simulink model "ITMBS_epushbtton_M1_Test_Harness"  (R2023a)
settings: Solver=FixedStepDiscrete  StartTime=0.0  StopTime=10  FixedStep=0.05  RelTol=1e-3
undefined symbols (not defined in the file or in its folder): sigbuilder_block
libraries: legoev3lib x2
settings Model: Creator=kevin  LastModifiedBy=Sachin K S

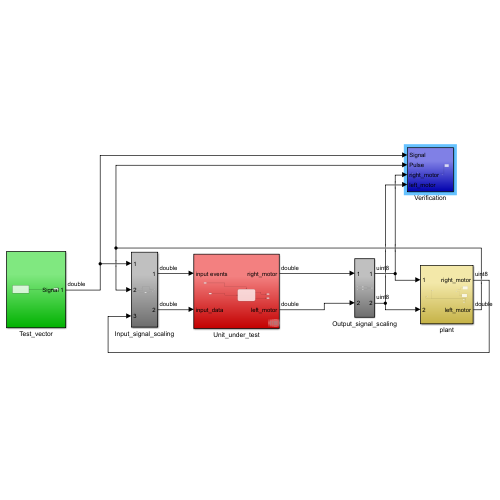
[thumbnail: Simulink's stored preview of the top-level diagram]
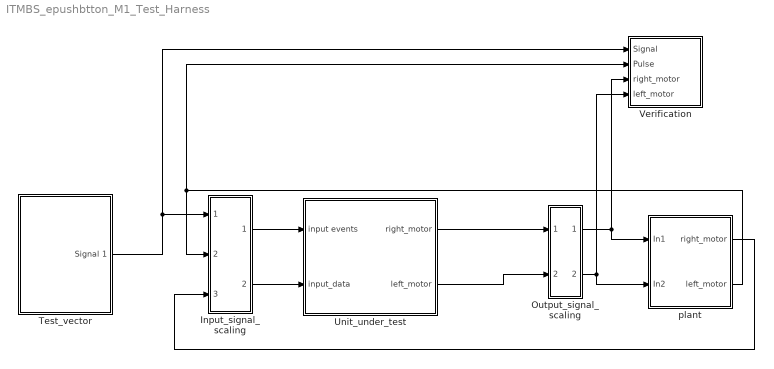
== system ITMBS_epushbtton_M1_Test_Harness ==
  Input_signal_scaling : Subsystem
  Output_signal_scaling : Subsystem
  Test_vector : Subsystem
  Unit_under_test : Subsystem
  Verification : Subsystem
  plant : Subsystem
  wires:
  Test_vector/1(Signal 1) -> Verification/1(Signal), Input_signal_scaling/1(In1)
  Unit_under_test/1(right_motor) -> Output_signal_scaling/1(In1)
  Output_signal_scaling/1(Out1) -> plant/1(In1), Verification/3(right_motor)
  plant/1(right_motor) -> Input_signal_scaling/3(In3)
  plant/2(left_motor) -> Verification/2(Pulse), Input_signal_scaling/2(In2)
  Unit_under_test/2(left_motor) -> Output_signal_scaling/2(In2)
  Input_signal_scaling/2(Out2) -> Unit_under_test/2(input_data)
  Input_signal_scaling/1(Out1) -> Unit_under_test/1(input events)
  Output_signal_scaling/2(Out2) -> plant/2(In2), Verification/4(left_motor)

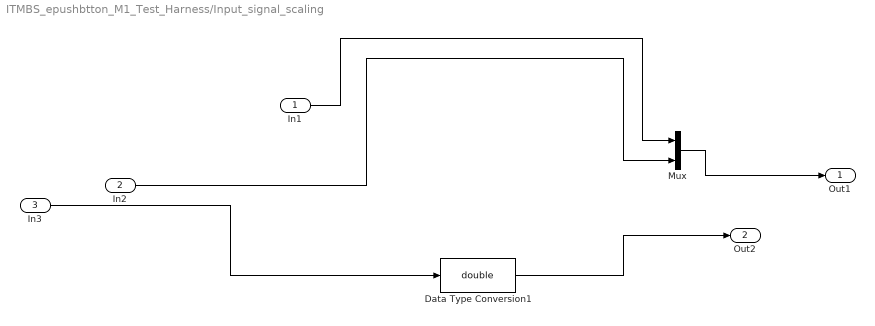
== system ITMBS_epushbtton_M1_Test_Harness/Input_signal_scaling ==
  In1 : Inport
  In2 : Inport  Port=2
  In3 : Inport  Port=3
  Data Type Conversion1 : DataTypeConversion  OutDataTypeStr=double  SaturateOnIntegerOverflow=off  RndMeth=Floor
  Mux : Mux  Inputs=2
  Out1 : Outport
  Out2 : Outport  Port=2
  wires:
  Mux/1 -> Out1/1
  Data Type Conversion1/1 -> Out2/1
  In2/1 -> Mux/2
  In1/1 -> Mux/1
  In3/1 -> Data Type Conversion1/1

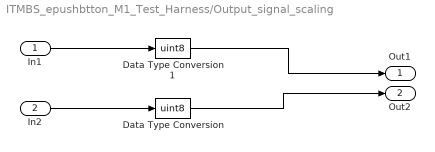
== system ITMBS_epushbtton_M1_Test_Harness/Output_signal_scaling ==
  In1 : Inport
  In2 : Inport  Port=2
  Data Type Conversion : DataTypeConversion  OutDataTypeStr=uint8  SaturateOnIntegerOverflow=off  RndMeth=Floor
  Data Type Conversion1 : DataTypeConversion  OutDataTypeStr=uint8  SaturateOnIntegerOverflow=off  RndMeth=Floor
  Out1 : Outport
  Out2 : Outport  Port=2
  wires:
  In1/1 -> Data Type Conversion1/1
  In2/1 -> Data Type Conversion/1
  Data Type Conversion/1 -> Out2/1
  Data Type Conversion1/1 -> Out1/1

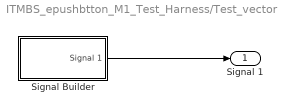
== system ITMBS_epushbtton_M1_Test_Harness/Test_vector ==
  Signal Builder : Subsystem  Tag=STV Subsys  LoadFcn=sigbuilder_block('load');  StartFcn=sigbuilder_block('start');  StopFcn=sigbuilder_block('stop');  ClipboardFcn=sigbuilder_block('clipboard');  mask(Sigbuilder block){tuvar=[0:10]}
      mask help: Simulink:masks:SigbuilderBlock_MD
      mask init:
      | if ~strcmp(get_param(bdroot(gcbh),'SimulationStatus'),'stopped') tuvar = sigbuilder_block('maskInit'); end
      settings: CopyFcn=sigbuilder_block('copy');  DeleteFcn=sigbuilder_block('delete');  ModelCloseFcn=sigbuilder_block('modelClose');  PreSaveFcn=sigbuilder_block('preSave');  PauseFcn=sigbuilder_block('pause');  ContinueFcn=sigbuilder_block('continue');  NameChangeFcn=sigbuilder_block('namechange');  OpenFcn=sigbuilder_block('open',[6 30 1012.5 447.75 ]);  CloseFcn=sigbuilder_block('close');
      mask Display: plot(0, 0, 100, 100,[2, 2, 32, 32, 2], [68, 8, 8, 68, 68],[32, 2], [38, 38], [32, 19, 2],[53, 60, 44], [32, 17, 17, 2],[16, 16, 31, 31]);txt = getActiveGroup(gcbh);text(2, 100, txt,'verticalAlignment', 'top');
  Signal 1 : Outport
  wires:
  Signal Builder/1(Signal 1) -> Signal 1/1

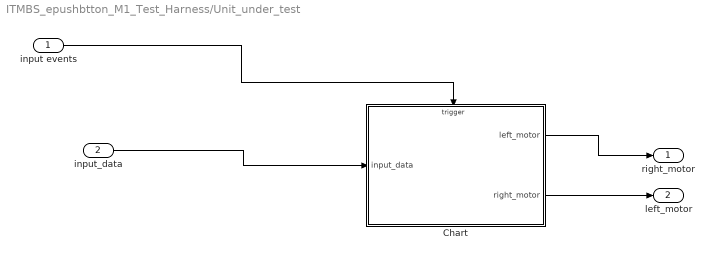
== system ITMBS_epushbtton_M1_Test_Harness/Unit_under_test ==
  input events : Inport
  input_data : Inport  Port=2
  Chart : Stateflow chart  TreatAsAtomicUnit=on
  right_motor : Outport
  left_motor : Outport  Port=2
  wires:
  input_data/1 -> Chart/1(input_data)
  input events/1 -> Chart/Trigger
  Chart/1(left_motor) -> right_motor/1
  Chart/2(right_motor) -> left_motor/1

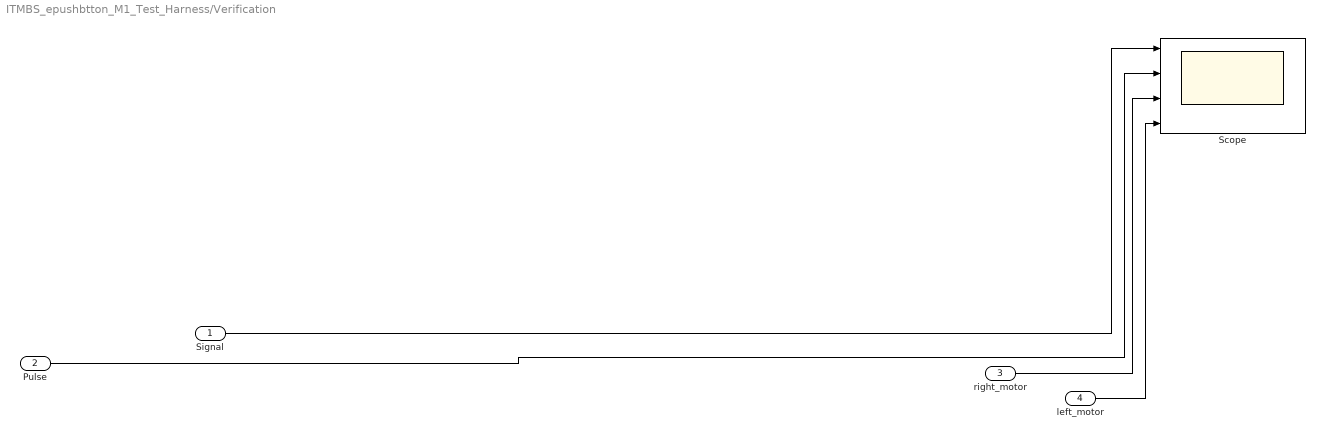
== system ITMBS_epushbtton_M1_Test_Harness/Verification ==
  Signal : Inport
  Pulse : Inport  Port=2
  right_motor : Inport  Port=3
  left_motor : Inport  Port=4
  Scope : Scope  NumInputPorts=4
  wires:
  Signal/1 -> Scope/1
  Pulse/1 -> Scope/2
  left_motor/1 -> Scope/4
  right_motor/1 -> Scope/3

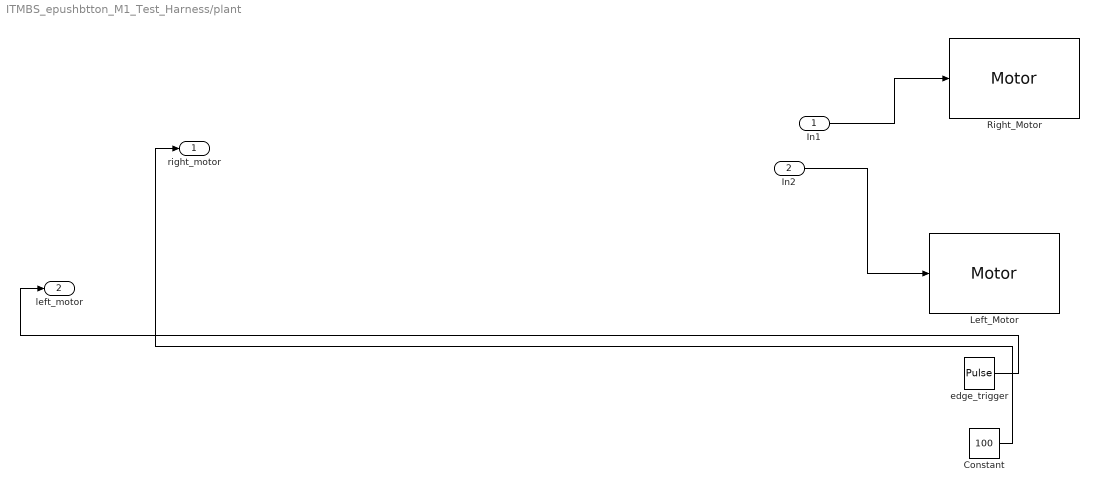
== system ITMBS_epushbtton_M1_Test_Harness/plant ==
  In1 : Inport
  In2 : Inport  Port=2
  Constant : Constant  Value=100  OutDataTypeStr=uint8
  Left_Motor : legoev3lib/Motor  sportNumber=B  sstopAction=Brake
  Right_Motor : legoev3lib/Motor  sportNumber=A  sstopAction=Brake
  edge_trigger : DiscretePulseGenerator  Period=3  PulseWidth=2  SampleTime=0.05
  right_motor : Outport
  left_motor : Outport  Port=2
  wires:
  In2/1 -> Left_Motor/1
  In1/1 -> Right_Motor/1
  Constant/1 -> right_motor/1
  edge_trigger/1 -> left_motor/1

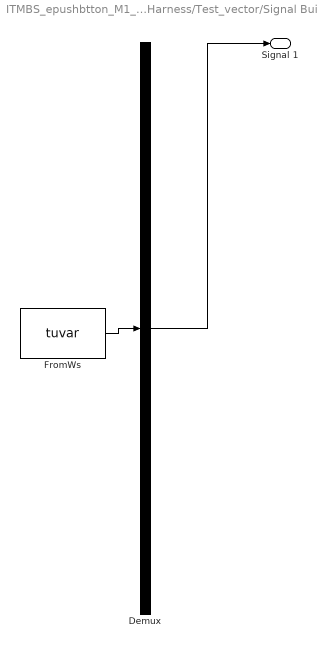
== system ITMBS_epushbtton_M1_Test_Harness/Test_vector/Signal Builder ==
  Demux : Demux  Tag=STV Demux  Outputs=1
      settings: DisplayOption=none
  FromWs : FromWorkspace  Tag=STV FromWs  VariableName=tuvar
      SigBuilderData=|
      | common.afterFinalStr = 'Extrapolate'
      | common.sampleTime = 0
      | dataSet.timeRange = [0 10]
      | dataSet.name = 'Group 1'
      | sbobj.Groups.Name = 'Group 1'
      | sbobj.Groups.Signals.Name = 'Signal 1'
      | sbobj.Groups.Signals.XData = [0 0.77 0.77 0.99 0.99 2.4 2.4 2.51 2.51 2.79 2.79 2.97 2.97 10]
      | sbobj.Groups.Signals.YData = [0 0 1 1 0 -0.005 0.995 1 0 0 0.995 0.995 0 0]
  Signal 1 : Outport  Tag=STV Outport
  wires:
  Demux/1 -> Signal 1/1
  FromWs/1 -> Demux/1

== stateflow chart ITMBS_epushbtton_M1_Test_Harness/Unit_under_test/Chart ==
  settings: executeAtInitialization=1
  state start
    right_motor = input_data;
    left_motor = input_data;
  state stop
    entry:
    right_motor=0;
    left_motor=0;
    c=0;
  (default) -> start
  start -> stop : pushbutton_event_input||(after(1.95,sec))
  (junction 38) -> start [order 1] : [c==2]
  stop -> (junction 36)
  (junction 36) -> (junction 37) [order 1] : [pushbutton_event_input]
  (junction 36) -> (junction 38) [order 2]
  (junction 37) -> (junction 39) : {c= c+1;}
  (junction 39) -> (junction 38)
  (junction 38) -> (junction 53) [order 2]
  data: input_data input; c local; left_motor output; right_motor output
  events: pushbutton_event_input input RISING_EDGE_EVENT; trigger input RISING_EDGE_EVENT
